simulink model "Par7InDegree"  (R2018a)
settings: Solver=VariableStepAuto  StartTime=0.0  StopTime=100  RelTol=1e-3
settings Model: Creator=wangluo  LastModifiedBy=wangluo

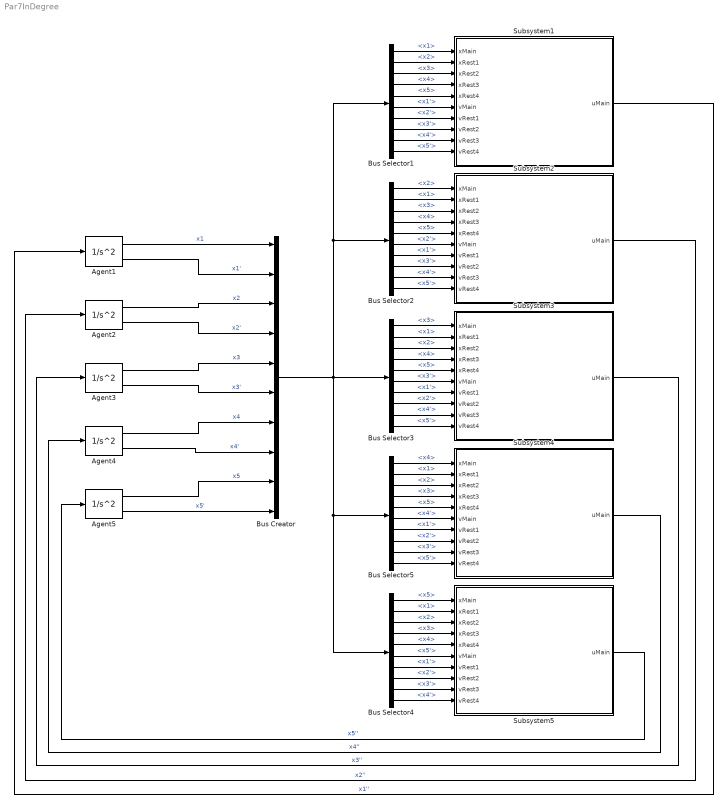
== system Par7InDegree ==
  Agent1 : SecondOrderIntegrator  ICX=100  ICDXDT=4
  Agent2 : SecondOrderIntegrator  ICX=150  ICDXDT=8
  Agent3 : SecondOrderIntegrator  ICX=250  ICDXDT=15
  Agent4 : SecondOrderIntegrator  ICX=200  ICDXDT=10
  Agent5 : SecondOrderIntegrator  ICX=300  ICDXDT=7
  Bus Creator : BusCreator  Inputs=10
  Bus Selector1 : BusSelector  OutputSignals=x1,x2,x3,x4,x5,x1',x2',x3',x4',x5'
  Bus Selector2 : BusSelector  OutputSignals=x2,x1,x3,x4,x5,x2',x1',x3',x4',x5'
  Bus Selector3 : BusSelector  OutputSignals=x3,x1,x2,x4,x5,x3',x1',x2',x4',x5'
  Bus Selector4 : BusSelector  OutputSignals=x5,x1,x2,x3,x4,x5',x1',x2',x3',x4'
  Bus Selector5 : BusSelector  OutputSignals=x4,x1,x2,x3,x5,x4',x1',x2',x3',x5'
  Subsystem1 : Subsystem
  Subsystem2 : Subsystem
  Subsystem3 : Subsystem
  Subsystem4 : Subsystem
  Subsystem5 : Subsystem
  wires:
  Bus Creator/1 -> Bus Selector4/1, Bus Selector5/1, Bus Selector3/1, Bus Selector2/1, Bus Selector1/1
  Subsystem1/1(uMain) -> Agent1/1  "x1''"
  Subsystem2/1(uMain) -> Agent2/1  "x2''"
  Subsystem3/1(uMain) -> Agent3/1  "x3''"
  Subsystem4/1(uMain) -> Agent4/1  "x4''"
  Subsystem5/1(uMain) -> Agent5/1  "x5''"
  Bus Selector1/10 -> Subsystem1/10(vRest4)  "<x5'>"
  Bus Selector1/9 -> Subsystem1/9(vRest3)  "<x4'>"
  Bus Selector1/8 -> Subsystem1/8(vRest2)  "<x3'>"
  Bus Selector1/7 -> Subsystem1/7(vRest1)  "<x2'>"
  Bus Selector1/6 -> Subsystem1/6(vMain)  "<x1'>"
  Bus Selector1/5 -> Subsystem1/5(xRest4)  "<x5>"
  Bus Selector1/4 -> Subsystem1/4(xRest3)  "<x4>"
  Bus Selector1/3 -> Subsystem1/3(xRest2)  "<x3>"
  Bus Selector1/2 -> Subsystem1/2(xRest1)  "<x2>"
  Bus Selector1/1 -> Subsystem1/1(xMain)  "<x1>"
  Bus Selector2/3 -> Subsystem2/3(xRest2)  "<x3>"
  Bus Selector2/4 -> Subsystem2/4(xRest3)  "<x4>"
  Bus Selector2/5 -> Subsystem2/5(xRest4)  "<x5>"
  Bus Selector2/8 -> Subsystem2/8(vRest2)  "<x3'>"
  Bus Selector2/9 -> Subsystem2/9(vRest3)  "<x4'>"
  Bus Selector2/10 -> Subsystem2/10(vRest4)  "<x5'>"
  Bus Selector3/4 -> Subsystem3/4(xRest3)  "<x4>"
  Bus Selector3/5 -> Subsystem3/5(xRest4)  "<x5>"
  Bus Selector3/9 -> Subsystem3/9(vRest3)  "<x4'>"
  Bus Selector3/10 -> Subsystem3/10(vRest4)  "<x5'>"
  Bus Selector2/1 -> Subsystem2/1(xMain)  "<x2>"
  Bus Selector2/2 -> Subsystem2/2(xRest1)  "<x1>"
  Bus Selector2/6 -> Subsystem2/6(vMain)  "<x2'>"
  Bus Selector2/7 -> Subsystem2/7(vRest1)  "<x1'>"
  Bus Selector3/1 -> Subsystem3/1(xMain)  "<x3>"
  Bus Selector3/2 -> Subsystem3/2(xRest1)  "<x1>"
  Bus Selector3/3 -> Subsystem3/3(xRest2)  "<x2>"
  Bus Selector3/8 -> Subsystem3/8(vRest2)  "<x2'>"
  Bus Selector3/7 -> Subsystem3/7(vRest1)  "<x1'>"
  Bus Selector3/6 -> Subsystem3/6(vMain)  "<x3'>"
  Bus Selector4/1 -> Subsystem5/1(xMain)  "<x5>"
  Bus Selector4/2 -> Subsystem5/2(xRest1)  "<x1>"
  Bus Selector4/3 -> Subsystem5/3(xRest2)  "<x2>"
  Bus Selector4/4 -> Subsystem5/4(xRest3)  "<x3>"
  Bus Selector4/5 -> Subsystem5/5(xRest4)  "<x4>"
  Bus Selector4/6 -> Subsystem5/6(vMain)  "<x5'>"
  Bus Selector4/7 -> Subsystem5/7(vRest1)  "<x1'>"
  Bus Selector4/8 -> Subsystem5/8(vRest2)  "<x2'>"
  Bus Selector4/9 -> Subsystem5/9(vRest3)  "<x3'>"
  Bus Selector4/10 -> Subsystem5/10(vRest4)  "<x4'>"
  Bus Selector5/1 -> Subsystem4/1(xMain)  "<x4>"
  Bus Selector5/2 -> Subsystem4/2(xRest1)  "<x1>"
  Bus Selector5/3 -> Subsystem4/3(xRest2)  "<x2>"
  Bus Selector5/4 -> Subsystem4/4(xRest3)  "<x3>"
  Bus Selector5/5 -> Subsystem4/5(xRest4)  "<x5>"
  Bus Selector5/6 -> Subsystem4/6(vMain)  "<x4'>"
  Bus Selector5/7 -> Subsystem4/7(vRest1)  "<x1'>"
  Bus Selector5/8 -> Subsystem4/8(vRest2)  "<x2'>"
  Bus Selector5/9 -> Subsystem4/9(vRest3)  "<x3'>"
  Bus Selector5/10 -> Subsystem4/10(vRest4)  "<x5'>"
  Agent1/1 -> Bus Creator/1  "x1"
  Agent1/2 -> Bus Creator/2  "x1'"
  Agent2/1 -> Bus Creator/3  "x2"
  Agent2/2 -> Bus Creator/4  "x2'"
  Agent3/1 -> Bus Creator/5  "x3"
  Agent3/2 -> Bus Creator/6  "x3'"
  Agent4/1 -> Bus Creator/7  "x4"
  Agent4/2 -> Bus Creator/8  "x4'"
  Agent5/1 -> Bus Creator/9  "x5"
  Agent5/2 -> Bus Creator/10  "x5'"

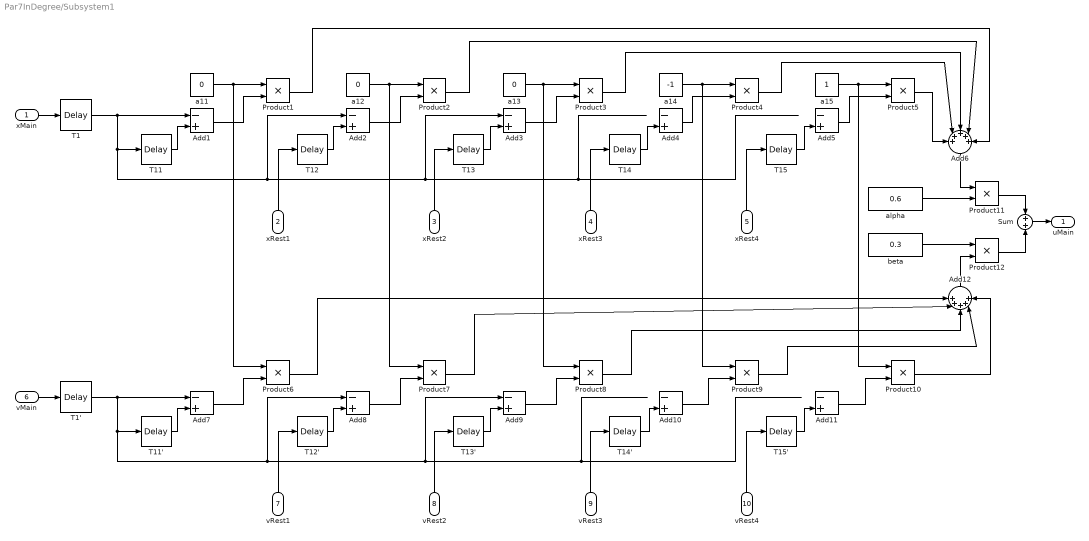
== system Par7InDegree/Subsystem1 ==
  xMain : Inport
  xRest1 : Inport  Port=2
  xRest2 : Inport  Port=3
  xRest3 : Inport  Port=4
  xRest4 : Inport  Port=5
  vMain : Inport  Port=6
  vRest1 : Inport  Port=7
  vRest2 : Inport  Port=8
  vRest3 : Inport  Port=9
  vRest4 : Inport  Port=10
  Add{1..5,7..11} (10 alike) : Sum  Inputs=-+
  Add12 : Sum  Inputs=+++++
  Add6 : Sum  Inputs=+++++
  Product{1..12} (12 alike) : Product
  Sum : Sum
  T{1,11..15} (6 alike) : TransportDelay  DelayTime=0
  T1' : TransportDelay  DelayTime=0
  T11' : TransportDelay  DelayTime=0
  T12' : TransportDelay  DelayTime=0
  T13' : TransportDelay  DelayTime=0
  T14' : TransportDelay  DelayTime=0
  T15' : TransportDelay  DelayTime=0
  a11 : Constant  Value=0
  a12 : Constant  Value=0
  a13 : Constant  Value=0
  a14 : Constant  Value=-1
  a15 : Constant
  alpha : Constant  Value=0.6
  beta : Constant  Value=0.3
  uMain : Outport
  wires:
  Add1/1 -> Product1/2
  T11/1 -> Add1/2
  T12/1 -> Add2/2
  Add2/1 -> Product2/2
  T13/1 -> Add3/2
  Add3/1 -> Product3/2
  xMain/1 -> T1/1
  xRest4/1 -> T15/1
  xRest3/1 -> T14/1
  xRest2/1 -> T13/1
  xRest1/1 -> T12/1
  Add6/1 -> Product11/1
  a11/1 -> Product6/1, Product1/1
  vMain/1 -> T1'/1
  a12/1 -> Product7/1, Product2/1
  Product9/1 -> Add12/4
  T11'/1 -> Add7/2
  vRest2/1 -> T13'/1
  Add9/1 -> Product8/2
  a14/1 -> Product9/1, Product4/1
  Add7/1 -> Product6/2
  Product10/1 -> Add12/5
  Product7/1 -> Add12/2
  a15/1 -> Product10/1, Product5/1
  T12'/1 -> Add8/2
  Add8/1 -> Product7/2
  T13'/1 -> Add9/2
  a13/1 -> Product8/1, Product3/1
  Product8/1 -> Add12/3
  vRest3/1 -> T14'/1
  vRest1/1 -> T12'/1
  vRest4/1 -> T15'/1
  Product6/1 -> Add12/1
  beta/1 -> Product12/1
  Add12/1 -> Product12/2
  alpha/1 -> Product11/2
  Product5/1 -> Add6/1
  Product4/1 -> Add6/2
  Product3/1 -> Add6/3
  Product2/1 -> Add6/4
  Product1/1 -> Add6/5
  Sum/1 -> uMain/1
  Product11/1 -> Sum/1
  Product12/1 -> Sum/2
  T1/1 -> Add1/1, T11/1, Add3/1, Add2/1
  T1'/1 -> Add7/1, T11'/1, Add9/1, Add8/1
  T14/1 -> Add4/2
  Add4/1 -> Product4/2
  T15/1 -> Add5/2
  Add5/1 -> Product5/2
  Add11/1 -> Product10/2
  T15'/1 -> Add11/2
  T14'/1 -> Add10/2
  Add10/1 -> Product9/2

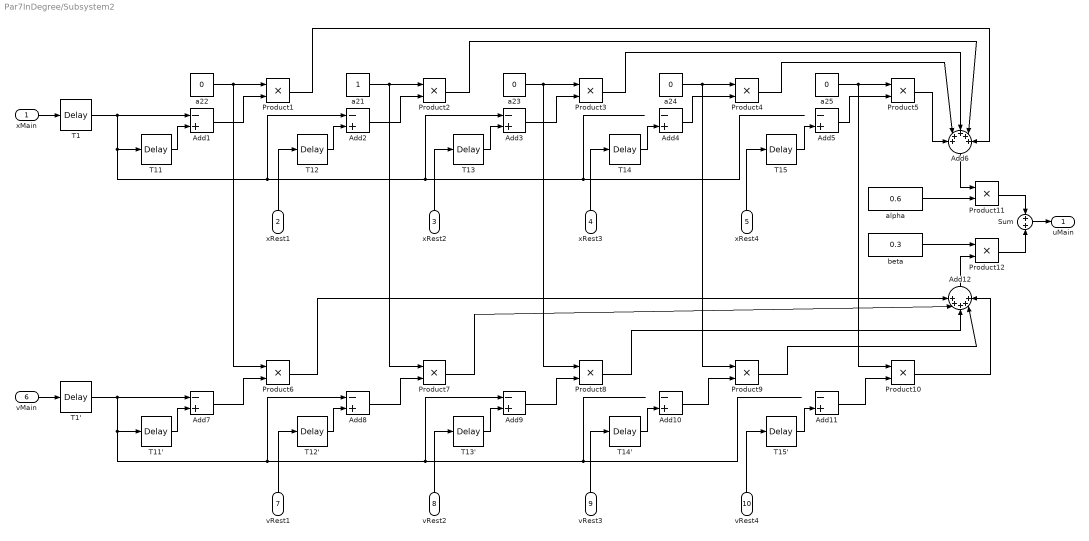
== system Par7InDegree/Subsystem2 ==
  xMain : Inport
  xRest1 : Inport  Port=2
  xRest2 : Inport  Port=3
  xRest3 : Inport  Port=4
  xRest4 : Inport  Port=5
  vMain : Inport  Port=6
  vRest1 : Inport  Port=7
  vRest2 : Inport  Port=8
  vRest3 : Inport  Port=9
  vRest4 : Inport  Port=10
  Add{1..5,7..11} (10 alike) : Sum  Inputs=-+
  Add12 : Sum  Inputs=+++++
  Add6 : Sum  Inputs=+++++
  Product{1..12} (12 alike) : Product
  Sum : Sum
  T{1,11..15} (6 alike) : TransportDelay  DelayTime=0
  T1' : TransportDelay  DelayTime=0
  T11' : TransportDelay  DelayTime=0
  T12' : TransportDelay  DelayTime=0
  T13' : TransportDelay  DelayTime=0
  T14' : TransportDelay  DelayTime=0
  T15' : TransportDelay  DelayTime=0
  a21 : Constant
  a{22..25} (4 alike) : Constant  Value=0
  alpha : Constant  Value=0.6
  beta : Constant  Value=0.3
  uMain : Outport
  wires:
  Add1/1 -> Product1/2
  T11/1 -> Add1/2
  T12/1 -> Add2/2
  Add2/1 -> Product2/2
  T13/1 -> Add3/2
  Add3/1 -> Product3/2
  xMain/1 -> T1/1
  xRest4/1 -> T15/1
  xRest3/1 -> T14/1
  xRest2/1 -> T13/1
  xRest1/1 -> T12/1
  Add6/1 -> Product11/1
  a22/1 -> Product6/1, Product1/1
  vMain/1 -> T1'/1
  a21/1 -> Product7/1, Product2/1
  Product9/1 -> Add12/4
  T11'/1 -> Add7/2
  vRest2/1 -> T13'/1
  Add9/1 -> Product8/2
  a24/1 -> Product9/1, Product4/1
  Add7/1 -> Product6/2
  Product10/1 -> Add12/5
  Product7/1 -> Add12/2
  a25/1 -> Product10/1, Product5/1
  T12'/1 -> Add8/2
  Add8/1 -> Product7/2
  T13'/1 -> Add9/2
  a23/1 -> Product8/1, Product3/1
  Product8/1 -> Add12/3
  vRest3/1 -> T14'/1
  vRest1/1 -> T12'/1
  vRest4/1 -> T15'/1
  Product6/1 -> Add12/1
  beta/1 -> Product12/1
  Add12/1 -> Product12/2
  alpha/1 -> Product11/2
  Product5/1 -> Add6/1
  Product4/1 -> Add6/2
  Product3/1 -> Add6/3
  Product2/1 -> Add6/4
  Product1/1 -> Add6/5
  Sum/1 -> uMain/1
  Product11/1 -> Sum/1
  Product12/1 -> Sum/2
  T1/1 -> Add1/1, T11/1, Add3/1, Add2/1
  T1'/1 -> Add7/1, T11'/1, Add9/1, Add8/1
  T14'/1 -> Add10/2
  T15'/1 -> Add11/2
  Add11/1 -> Product10/2
  Add10/1 -> Product9/2
  Add4/1 -> Product4/2
  T14/1 -> Add4/2
  T15/1 -> Add5/2
  Add5/1 -> Product5/2

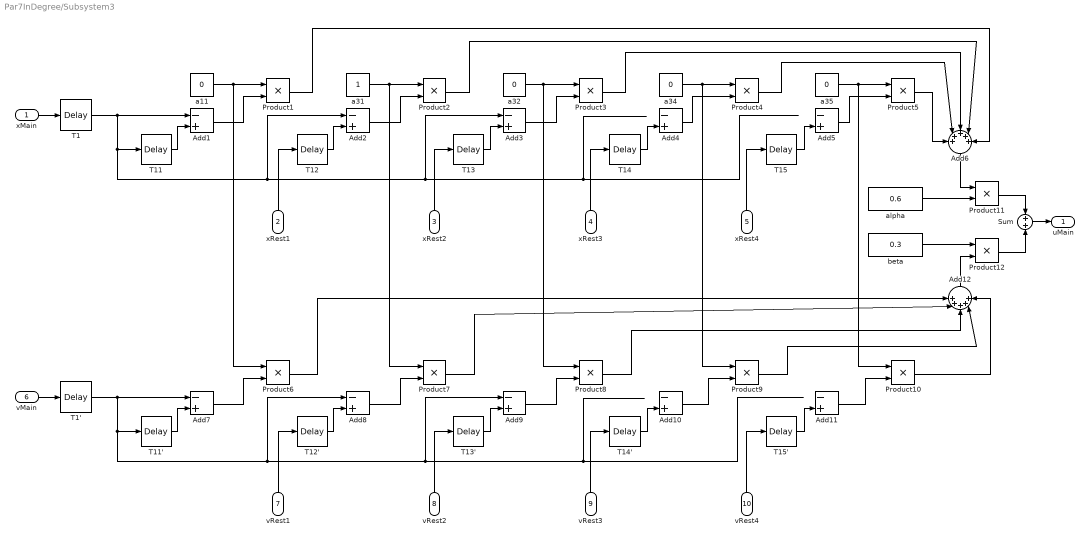
== system Par7InDegree/Subsystem3 ==
  xMain : Inport
  xRest1 : Inport  Port=2
  xRest2 : Inport  Port=3
  xRest3 : Inport  Port=4
  xRest4 : Inport  Port=5
  vMain : Inport  Port=6
  vRest1 : Inport  Port=7
  vRest2 : Inport  Port=8
  vRest3 : Inport  Port=9
  vRest4 : Inport  Port=10
  Add{1..5,7..11} (10 alike) : Sum  Inputs=-+
  Add12 : Sum  Inputs=+++++
  Add6 : Sum  Inputs=+++++
  Product{1..12} (12 alike) : Product
  Sum : Sum
  T{1,11..15} (6 alike) : TransportDelay  DelayTime=0
  T1' : TransportDelay  DelayTime=0
  T11' : TransportDelay  DelayTime=0
  T12' : TransportDelay  DelayTime=0
  T13' : TransportDelay  DelayTime=0
  T14' : TransportDelay  DelayTime=0
  T15' : TransportDelay  DelayTime=0
  a{11,32,34..35} (4 alike) : Constant  Value=0
  a31 : Constant
  alpha : Constant  Value=0.6
  beta : Constant  Value=0.3
  uMain : Outport
  wires:
  Add1/1 -> Product1/2
  T11/1 -> Add1/2
  T12/1 -> Add2/2
  Add2/1 -> Product2/2
  T13/1 -> Add3/2
  Add3/1 -> Product3/2
  xMain/1 -> T1/1
  xRest4/1 -> T15/1
  xRest3/1 -> T14/1
  xRest2/1 -> T13/1
  xRest1/1 -> T12/1
  Add6/1 -> Product11/1
  a11/1 -> Product6/1, Product1/1
  vMain/1 -> T1'/1
  a31/1 -> Product7/1, Product2/1
  Product9/1 -> Add12/4
  T11'/1 -> Add7/2
  vRest2/1 -> T13'/1
  Add9/1 -> Product8/2
  a34/1 -> Product9/1, Product4/1
  Add7/1 -> Product6/2
  Product10/1 -> Add12/5
  Product7/1 -> Add12/2
  a35/1 -> Product10/1, Product5/1
  T12'/1 -> Add8/2
  Add8/1 -> Product7/2
  T13'/1 -> Add9/2
  a32/1 -> Product8/1, Product3/1
  Product8/1 -> Add12/3
  vRest3/1 -> T14'/1
  vRest1/1 -> T12'/1
  vRest4/1 -> T15'/1
  Product6/1 -> Add12/1
  beta/1 -> Product12/1
  Add12/1 -> Product12/2
  alpha/1 -> Product11/2
  Product5/1 -> Add6/1
  Product4/1 -> Add6/2
  Product3/1 -> Add6/3
  Product2/1 -> Add6/4
  Product1/1 -> Add6/5
  Sum/1 -> uMain/1
  Product11/1 -> Sum/1
  Product12/1 -> Sum/2
  T1/1 -> Add1/1, T11/1, Add3/1, Add2/1
  T1'/1 -> Add7/1, T11'/1, Add9/1, Add8/1
  T15/1 -> Add5/2
  Add5/1 -> Product5/2
  Add11/1 -> Product10/2
  T15'/1 -> Add11/2
  Add10/1 -> Product9/2
  T14'/1 -> Add10/2
  Add4/1 -> Product4/2
  T14/1 -> Add4/2

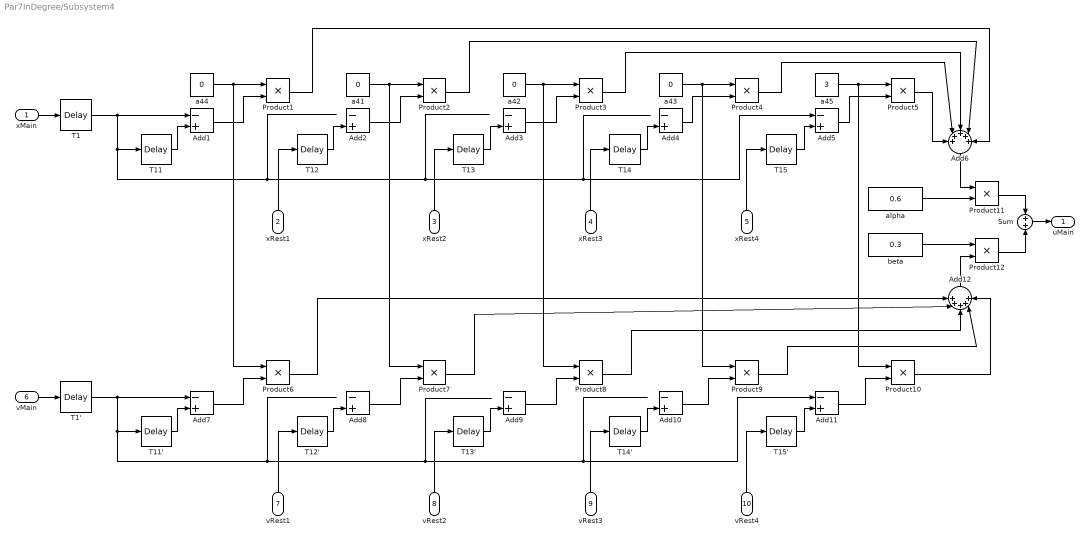
== system Par7InDegree/Subsystem4 ==
  xMain : Inport
  xRest1 : Inport  Port=2
  xRest2 : Inport  Port=3
  xRest3 : Inport  Port=4
  xRest4 : Inport  Port=5
  vMain : Inport  Port=6
  vRest1 : Inport  Port=7
  vRest2 : Inport  Port=8
  vRest3 : Inport  Port=9
  vRest4 : Inport  Port=10
  Add{1..5,7..11} (10 alike) : Sum  Inputs=-+
  Add12 : Sum  Inputs=+++++
  Add6 : Sum  Inputs=+++++
  Product{1..12} (12 alike) : Product
  Sum : Sum
  T{1,11..15} (6 alike) : TransportDelay  DelayTime=0
  T1' : TransportDelay  DelayTime=0
  T11' : TransportDelay  DelayTime=0
  T12' : TransportDelay  DelayTime=0
  T13' : TransportDelay  DelayTime=0
  T14' : TransportDelay  DelayTime=0
  T15' : TransportDelay  DelayTime=0
  a{41..44} (4 alike) : Constant  Value=0
  a45 : Constant  Value=3
  alpha : Constant  Value=0.6
  beta : Constant  Value=0.3
  uMain : Outport
  wires:
  Add1/1 -> Product1/2
  T11/1 -> Add1/2
  T12/1 -> Add2/2
  Add2/1 -> Product2/2
  T13/1 -> Add3/2
  Add3/1 -> Product3/2
  xMain/1 -> T1/1
  xRest4/1 -> T15/1
  xRest3/1 -> T14/1
  xRest2/1 -> T13/1
  xRest1/1 -> T12/1
  Add6/1 -> Product11/1
  a44/1 -> Product6/1, Product1/1
  vMain/1 -> T1'/1
  a41/1 -> Product7/1, Product2/1
  Product9/1 -> Add12/4
  T11'/1 -> Add7/2
  vRest2/1 -> T13'/1
  Add9/1 -> Product8/2
  a43/1 -> Product9/1, Product4/1
  Add7/1 -> Product6/2
  Product10/1 -> Add12/5
  Product7/1 -> Add12/2
  a45/1 -> Product10/1, Product5/1
  T12'/1 -> Add8/2
  Add8/1 -> Product7/2
  T13'/1 -> Add9/2
  a42/1 -> Product8/1, Product3/1
  Product8/1 -> Add12/3
  vRest3/1 -> T14'/1
  vRest1/1 -> T12'/1
  vRest4/1 -> T15'/1
  Product6/1 -> Add12/1
  beta/1 -> Product12/1
  Add12/1 -> Product12/2
  alpha/1 -> Product11/2
  Product5/1 -> Add6/1
  Product4/1 -> Add6/2
  Product3/1 -> Add6/3
  Product2/1 -> Add6/4
  Product1/1 -> Add6/5
  Sum/1 -> uMain/1
  Product11/1 -> Sum/1
  Product12/1 -> Sum/2
  T1/1 -> Add1/1, T11/1, Add5/1
  T1'/1 -> Add7/1, T11'/1, Add11/1
  T15/1 -> Add5/2
  Add5/1 -> Product5/2
  T14/1 -> Add4/2
  Add4/1 -> Product4/2
  T15'/1 -> Add11/2
  Add11/1 -> Product10/2
  T14'/1 -> Add10/2
  Add10/1 -> Product9/2

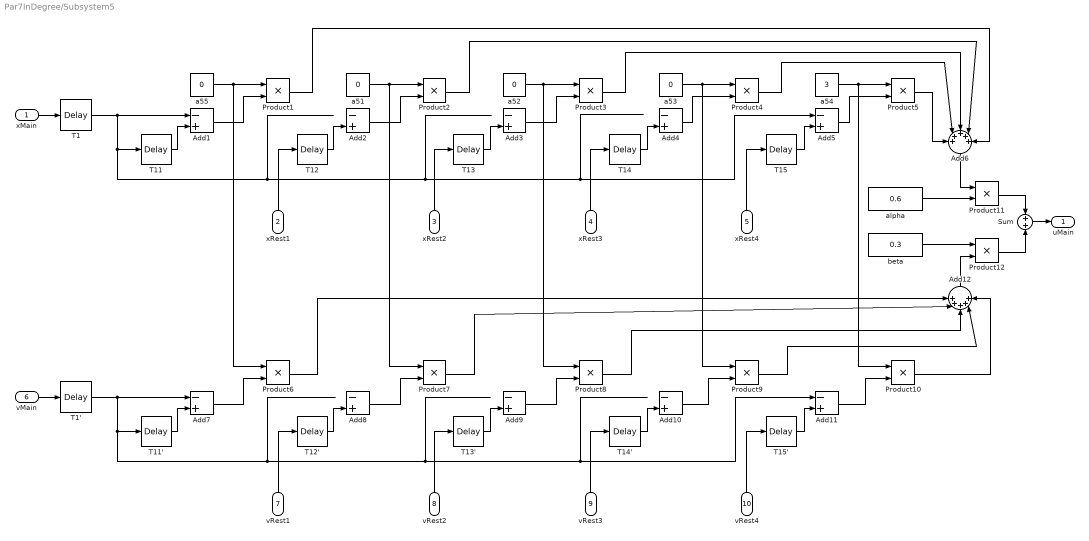
== system Par7InDegree/Subsystem5 ==
  xMain : Inport
  xRest1 : Inport  Port=2
  xRest2 : Inport  Port=3
  xRest3 : Inport  Port=4
  xRest4 : Inport  Port=5
  vMain : Inport  Port=6
  vRest1 : Inport  Port=7
  vRest2 : Inport  Port=8
  vRest3 : Inport  Port=9
  vRest4 : Inport  Port=10
  Add{1..5,7..11} (10 alike) : Sum  Inputs=-+
  Add12 : Sum  Inputs=+++++
  Add6 : Sum  Inputs=+++++
  Product{1..12} (12 alike) : Product
  Sum : Sum
  T{1,11..15} (6 alike) : TransportDelay  DelayTime=0
  T1' : TransportDelay  DelayTime=0
  T11' : TransportDelay  DelayTime=0
  T12' : TransportDelay  DelayTime=0
  T13' : TransportDelay  DelayTime=0
  T14' : TransportDelay  DelayTime=0
  T15' : TransportDelay  DelayTime=0
  a{51..53,55} (4 alike) : Constant  Value=0
  a54 : Constant  Value=3
  alpha : Constant  Value=0.6
  beta : Constant  Value=0.3
  uMain : Outport
  wires:
  Add1/1 -> Product1/2
  T11/1 -> Add1/2
  T12/1 -> Add2/2
  Add2/1 -> Product2/2
  T13/1 -> Add3/2
  Add3/1 -> Product3/2
  xMain/1 -> T1/1
  xRest4/1 -> T15/1
  xRest3/1 -> T14/1
  xRest2/1 -> T13/1
  xRest1/1 -> T12/1
  Add6/1 -> Product11/1
  a55/1 -> Product6/1, Product1/1
  vMain/1 -> T1'/1
  a51/1 -> Product7/1, Product2/1
  Product9/1 -> Add12/4
  T11'/1 -> Add7/2
  vRest2/1 -> T13'/1
  Add9/1 -> Product8/2
  a53/1 -> Product9/1, Product4/1
  Add7/1 -> Product6/2
  Product10/1 -> Add12/5
  Product7/1 -> Add12/2
  a54/1 -> Product10/1, Product5/1
  T12'/1 -> Add8/2
  Add8/1 -> Product7/2
  T13'/1 -> Add9/2
  a52/1 -> Product8/1, Product3/1
  Product8/1 -> Add12/3
  vRest3/1 -> T14'/1
  vRest1/1 -> T12'/1
  vRest4/1 -> T15'/1
  Product6/1 -> Add12/1
  beta/1 -> Product12/1
  Add12/1 -> Product12/2
  alpha/1 -> Product11/2
  Product5/1 -> Add6/1
  Product4/1 -> Add6/2
  Product3/1 -> Add6/3
  Product2/1 -> Add6/4
  Product1/1 -> Add6/5
  Sum/1 -> uMain/1
  Product11/1 -> Sum/1
  Product12/1 -> Sum/2
  T1/1 -> Add1/1, T11/1, Add5/1
  T1'/1 -> Add7/1, T11'/1, Add11/1
  T14/1 -> Add4/2
  Add4/1 -> Product4/2
  T15/1 -> Add5/2
  Add5/1 -> Product5/2
  T14'/1 -> Add10/2
  Add10/1 -> Product9/2
  T15'/1 -> Add11/2
  Add11/1 -> Product10/2
